simulink model "sim_arm_sfbk_servo"  (R2019b)
settings: Solver=ode4  StartTime=0.0  StopTime=2  FixedStep=0.001  RelTol=1e-3
values from neighbouring files (symbols this model uses):
  A = [  0         1 ... (first row only)    [example_09_02_sym.m]    (also in example_09_04.m = [  0    1; example_09_04_sym.m = [  0    1; example_09_05_sym.m = [ a11  0; example_09_06_sym.m = [ a11  0)
  B = [  0 ... (first row only)    [example_09_02_sym.m]    (also in example_09_05_sym.m = [ 0; example_09_06_sym.m = [ b1; example_09_07.m = [ 0; example_09_07_sym.m = [ 0)
  G = Ke(n+1)    [example_09_12.m]    (also in example_09_12_R2015a.m; example_09_12_R2018a.m)
  K = - acker(A,B,p)    [example_09_07.m]    (also in example_09_07_sym.m = sym('k',[1 n],'real'); example_09_07b.m; example_09_07b_R2015a.m; example_09_07b_R2018a.m)
settings Model: Creator=kawata  LastModifiedBy=kawata
settings DataIOCC: ReturnWorkspaceOutputs=off
settings DebuggingCC: ArithmeticOperatorsInVariantConditions=warning
settings SFSimCC: SimUseLocalCustomCode=off  CustomCodeUndefinedFunction=UseInterfaceOnly
settings RTWCC: RTWUseLocalCustomCode=off

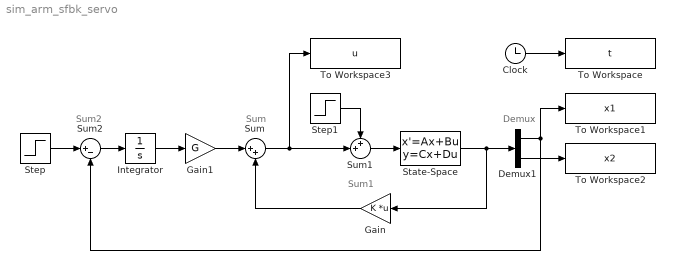
== system sim_arm_sfbk_servo ==
  note: Demux
  note: Sum
  note: Sum1
  note: Sum2
  Clock : Clock
  Demux1 : Demux  Outputs=2
  Gain : Gain  Gain=K  Multiplication=Matrix(K*u)
  Gain1 : Gain  Gain=G
  Integrator : Integrator
  State-Space : StateSpace  A=A  B=B  C=eye(2)  D=zeros(2,1)  InitialCondition=0
  Step : Step  Time=0  SampleTime=0
  Step1 : Step  SampleTime=0
  Sum : Sum  Inputs=|++
  Sum1 : Sum  Inputs=++|
  Sum2 : Sum  Inputs=|+-
  To Workspace : ToWorkspace  VariableName=t  SampleTime=-1
  To Workspace1 : ToWorkspace  VariableName=x1  SampleTime=-1
  To Workspace2 : ToWorkspace  VariableName=x2  SampleTime=-1
  To Workspace3 : ToWorkspace  VariableName=u  SampleTime=-1
  wires:
  State-Space/1 -> Gain/1, Demux1/1
  Clock/1 -> To Workspace/1
  Demux1/1 -> To Workspace1/1, Sum2/2
  Demux1/2 -> To Workspace2/1
  Gain/1 -> Sum/2
  Sum1/1 -> State-Space/1
  Sum/1 -> To Workspace3/1, Sum1/2
  Step1/1 -> Sum1/1
  Step/1 -> Sum2/1
  Sum2/1 -> Integrator/1
  Integrator/1 -> Gain1/1
  Gain1/1 -> Sum/1
